simulink model "dspsdadc_sg_LL03_IIR_DC_rem"  (R2016b)
settings: Solver=ode5  StartTime=0.0  StopTime=2*pi*200000/2.4e6  MaxStep=1/512000  RelTol=1e-3  AbsTol=1e-6
PreLoadFcn:
  | input_rate = 2.5e6;
  | input_period = 1/input_rate;
  | decimation_factor = 64;
  | 
  | 
  | ila_PDM_data = read_vectored_ILA_PDM_capture('.\ILA_capture\iladata_A440_vectors_1024.csv');
  | % ila_PDM_data = read_vectored_ILA_PDM_capture('.\ILA_capture\iladata_speech_vectors_1024.csv');
  | 
  | ila_data_struct.time = [];
  | ila_data_struct.signals.values = ila_PDM_data;
  | 
  | % Delay parameter for IIR DC-removal filter
  | D= 256;
StopFcn:
  | p = audioplayer(squeeze(simout_demodulated_SG.Data), input_rate/decimation_factor);
  | play(p, [1 (get(p, 'SampleRate') * 1)]);
  | 
  | p = audioplayer(squeeze(simout_demodulated_FP.Data), input_rate/decimation_factor);
  | play(p, [1 (get(p, 'SampleRate') * 1)]);
undefined symbols (not defined in the file or in its folder): xlfda_numerator
libraries: xbsIndex_r4 x30, dspmlti4 x2, simulink x1, dspmisc x1
settings Model: ExtModeTrigMode=oneshot  ExtModeArmWhenConnect=off  ExtModeAutoUpdateStatusClock=off  Creator=The MathWorks Inc.  LastModifiedBy=Luc
settings DataIOCC: SaveFormat=Array  SaveOutput=off  SaveTime=off  SignalLoggingName=logsOut
settings OptimizationCC: BlockReduction=off  BooleanDataType=off  ExpressionDepthLimit=2147483647  RollThreshold=2  InitFltsAndDblsToZero=on  EfficientMapNaN2IntZero=off  LifeSpan=inf
settings DebuggingCC: SaveWithParameterizedLinksMsg=none  UnderspecifiedInitializationDetection=Classic  MergeDetectMultiDrivingBlocksExec=none  SignalResolutionControl=TryResolveAllWithWarning  MultiTaskDSMMsg=warning  MultiTaskCondExecSysMsg=none  IntegerOverflowMsg=none  FcnCallInpInsideContextMsg=warning  StateNameClashWarn=warning  SFUnexpectedBacktrackingDiag=warning  SFNoUnconditionalDefaultTransitionDiag=warning  SFExecutionAtInitializationDiag=none  IntegerSaturationMsg=none
settings HardwareCC: ProdBitPerPointer=32  ProdBitPerSizeT=32  ProdBitPerPtrDiffT=32  ProdLargestAtomicFloat=None  ProdIntDivRoundTo=Undefined  ProdEndianess=Unspecified  ProdWordSize=32  ProdHWDeviceType=32-bit Generic  TargetUnknown=on
settings ModelReferenceCC: PropagateSignalLabelsOutOfModel=off
settings GRTTargetCC: TargetFcnLib=ansi_tfl_tmw.mat  TargetLangStandard=C89/C90 (ANSI)  GeneratePreprocessorConditionals=Disable all  CombineOutputUpdateFcns=off  GRTInterface=on
settings ConfigComp: CovMetricSettings=dw  CovHtmlReporting=on  CovSaveCumulativeToWorkspaceVar=on  CovSaveSingleToWorkspaceVar=on  CovExternalEMLEnable=off

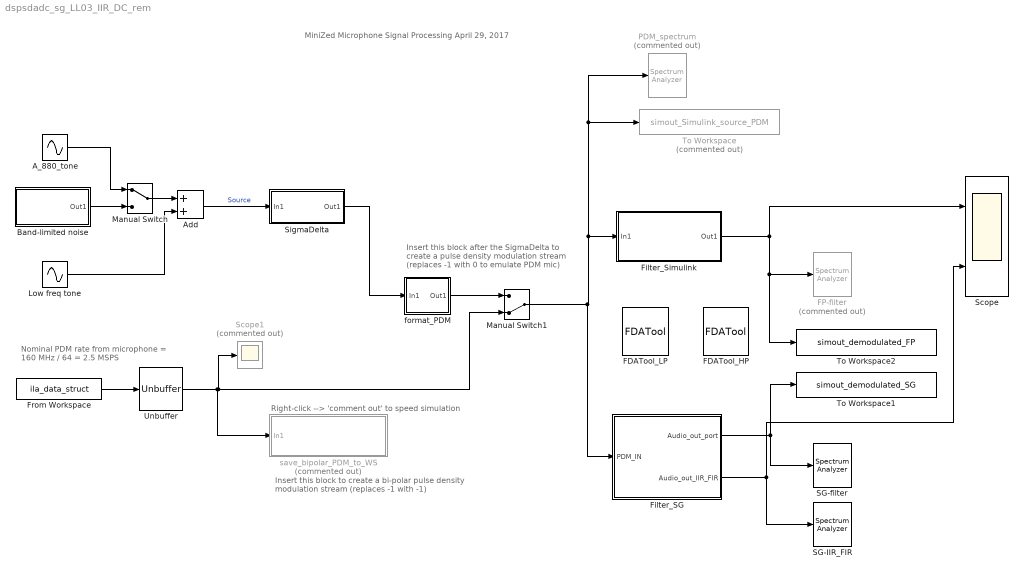
== system dspsdadc_sg_LL03_IIR_DC_rem ==
  note: Insert this block after the SigmaDelta to
      | create a pulse density modulation stream
      | (replaces -1 with 0 to emulate PDM mic)
  note: Insert this block to
      | create a bi-polar pulse density modulation stream
      | (replaces -1 with -1)
  note: Right-click --> 'comment out' to speed simulation
  note: Nominal PDM rate from microphone = 160 MHz / 64 = 2.5 MSPS
  note: MiniZed Microphone Signal Processing
      | April 29, 2017
  A_880_tone : Sin  Amplitude=0.5  Frequency=2*pi*880  SampleTime=input_period
  Add : Sum
  Band-limited noise : Subsystem
  FDATool_HP : xbsIndex_r4/FDATool  block_type=fdatool
      settings: infoedit=FDATool
  FDATool_LP : xbsIndex_r4/FDATool  block_type=fdatool
      settings: infoedit=FDATool
  FP-filter : SpectrumAnalyzer  Commented=on
  Filter_SG : Subsystem
  Filter_Simulink : Subsystem
  From Workspace : FromWorkspace  VariableName=ila_data_struct  OutDataTypeStr=double  SampleTime=input_period*1024  Interpolate=off  OutputAfterFinalValue=Cyclic repetition
  Low freq tone : Sin  Amplitude=0.0  Frequency=2*pi*5  SampleTime=input_period
  Manual Switch : ManualSwitch
  Manual Switch1 : ManualSwitch  CurrentSetting=0
  PDM_spectrum : SpectrumAnalyzer  Commented=on
  SG-IIR_FIR : SpectrumAnalyzer
  SG-filter : SpectrumAnalyzer
  Scope : Scope  NumInputPorts=2
  Scope1 : Scope  Commented=on
  SigmaDelta : Subsystem
  To Workspace : ToWorkspace  Commented=on  VariableName=simout_Simulink_source_PDM  SaveFormat=Timeseries  SampleTime=-1
  To Workspace1 : ToWorkspace  VariableName=simout_demodulated_SG  SaveFormat=Timeseries  SampleTime=-1
  To Workspace2 : ToWorkspace  VariableName=simout_demodulated_FP  SaveFormat=Timeseries  SampleTime=-1
  Unbuffer : Unbuffer  SampleBasedProcessing=Same as frame based
  format_PDM : Subsystem
  save_bipolar_PDM_to_WS : Subsystem  Commented=on
  wires:
  Add/1 -> SigmaDelta/1(In1)  "Source"
  Filter_SG/1(Audio_out_port) -> SG-filter/1, To Workspace1/1
  Filter_Simulink/1(Out1) -> Scope/1, To Workspace2/1, FP-filter/1
  Low freq tone/1 -> Add/2
  Manual Switch/1 -> Add/1
  A_880_tone/1 -> Manual Switch/1
  Band-limited noise/1(Out1) -> Manual Switch/2
  SigmaDelta/1(Out1) -> format_PDM/1(In1)
  Manual Switch1/1 -> PDM_spectrum/1, To Workspace/1, Filter_Simulink/1(In1), Filter_SG/1(PDM_IN)
  format_PDM/1(Out1) -> Manual Switch1/1
  From Workspace/1 -> Unbuffer/1
  Unbuffer/1 -> save_bipolar_PDM_to_WS/1(In1), Scope1/1, Manual Switch1/2
  Filter_SG/2(Audio_out_IIR_FIR) -> Scope/2, SG-IIR_FIR/1

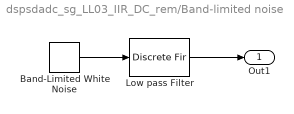
== system dspsdadc_sg_LL03_IIR_DC_rem/Band-limited noise ==
  Band-Limited White Noise : simulink/Sources/Band-Limited White Noise  Cov=[0.000001]  Ts=input_period  seed=[23341]
  Low pass Filter : DiscreteFir  Coefficients=xlfda_numerator([bdroot '/FDATool_LP'])
  Out1 : Outport
  wires:
  Band-Limited White Noise/1 -> Low pass Filter/1
  Low pass Filter/1 -> Out1/1

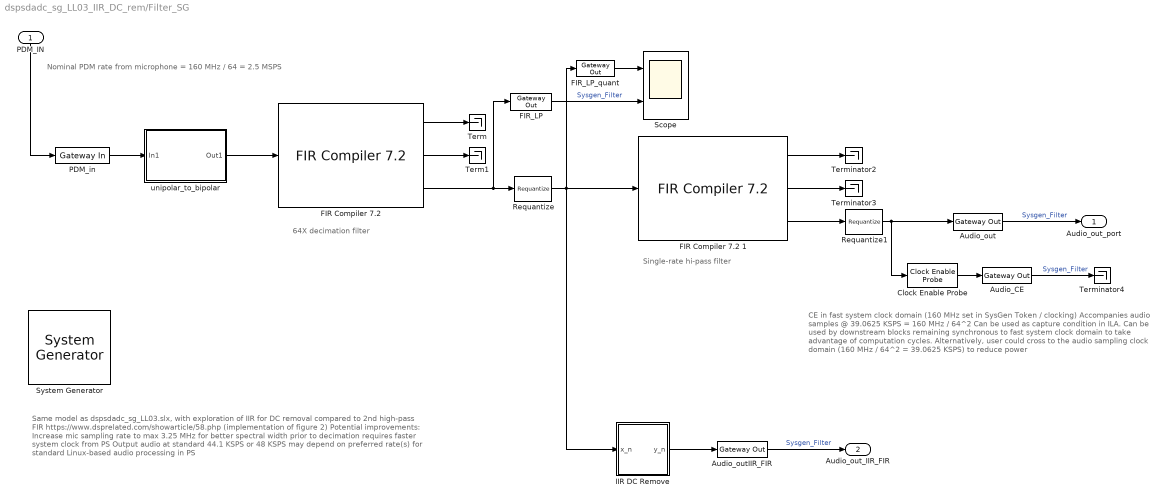
== system dspsdadc_sg_LL03_IIR_DC_rem/Filter_SG ==
  note: CE in fast system clock domain (160 MHz set in SysGen Token / clocking)
      | Accompanies audio samples @ 39.0625 KSPS = 160 MHz / 64^2
      |
      | Can be used as capture condition in ILA.
      |
      | Can be used by downstream blocks remaining synchronous to fast system clock domain to take advantage of computation cycles.
      |
      | Alternatively, user could cross to the audio sampling clock domain (160 MHz / 64^2 = 39.0625 KSPS) to reduce power
  note: Nominal PDM rate from microphone = 160 MHz / 64 = 2.5 MSPS
  note: 64X decimation filter
  note: Single-rate hi-pass filter
  note: Same model as dspsdadc_sg_LL03.slx, with exploration of IIR for DC removal compared to 2nd high-pass FIR
      | https://www.dsprelated.com/showarticle/58.php
      | (implementation of figure 2)
      |
      | Potential improvements:
      |
      | Increase mic sampling rate to max 3.25 MHz for better spectral width prior to decimation
      | requires faster system clock from PS
      | Output audio at standard 44.1 KSPS or 48 KSPS
      | may depend on preferred rate(s) for standard Linux-based audio processing in PS
  PDM_IN : Inport
  " System Generator" : xbsIndex_r4/ System Generator  Tag=genX  xilinxfamily=zynq  part=xc7z010  speed=-1  package=clg400  synthesis_tool=Vivado  clock_wrapper=Clock Enables  directory=C:/VivadoProjects/MiniZedBasic/SysGen/netlist  proj_type=Vivado  Synth_file=Vivado Synthesis Defaults  Impl_file=Vivado Implementation Defaults  testbench=off  simulink_period=1/(64*2.5e6)  sysclk_period=6.25  dcm_input_clock_period=10  incr_netlist=off  trim_vbits=Everywhere in SubSystem  dbl_ovrd=According to Block Masks  core_generation=According to Block Masks  run_coregen=off  deprecated_control=off  eval_field=0  block_type=sysgen
  Audio_CE : xbsIndex_r4/Gateway Out  inherit_from_input=off  hdl_port=on  rows=1  columns=1  UseAsDAC=off  DACChannel='1'  interface=None  automatic_assignment=on  address_offset=hex2dec('00')  intf_name=''  intf_description=''  timing_constraint=None  locs_specified=off  LOCs={}  io_standard={}  block_type=gatewayout
  Audio_out : xbsIndex_r4/Gateway Out  inherit_from_input=off  hdl_port=on  rows=1  columns=1  UseAsDAC=off  DACChannel='1'  interface=None  automatic_assignment=on  address_offset=hex2dec('00')  intf_name=''  intf_description=''  timing_constraint=None  locs_specified=off  LOCs={}  io_standard={}  block_type=gatewayout
  Audio_outIIR_FIR : xbsIndex_r4/Gateway Out  inherit_from_input=off  hdl_port=on  rows=1  columns=1  UseAsDAC=off  DACChannel='1'  interface=None  automatic_assignment=on  address_offset=hex2dec('00')  intf_name=''  intf_description=''  timing_constraint=None  locs_specified=off  LOCs={}  io_standard={}  block_type=gatewayout
  Clock Enable Probe : xbsIndex_r4/Clock Enable Probe  inherit_constraints=off  block_type=ceprobe
      settings: infoedit="Clock enable extractor.  Produces a Boolean output that mirrors the hardware clock enable associated with the input sample rate.<br><br>Hardware notes: in hardware this block costs nothing."
  "FIR Compiler 7.2 " : xbsIndex_r4/FIR Compiler 7.2   coefficientvector=xlfda_numerator([bdroot '/FDATool_LP'])* decimation_factor  coefficient_sets=1  coefficient_reload=off  filter_type=Decimation  rate_change_type=Integer  interpolation_rate=1  decimation_rate=decimation_factor  zero_pack_factor=1  channel_sequence=Basic  number_channels=1  pattern_list='P4-0,P4-1,P4-2,P4-3,P4-4'  number_paths=1  ratespecification=Maximum_Possible  sampleperiod=4096  hardwareoversamplingrate=1  coefficient_sign=Signed  quantization=Maximize_Dynamic_Range  coefficient_width=16  bestprecision=on  coefficient_fractional_bits=15  coefficient_structure=Symmetric  output_rounding_mode=Symmetric_Rounding_to_Infinity  output_width=21  filter_architecture=Systolic_Multiply_Accumulate  optimization_goal=Area  optimization_list='None'  data_buffer_type=Automatic  coefficient_buffer_type=Automatic  input_buffer_type=Automatic  output_buffer_type=Automatic  preference_for_other_storage=Automatic  multi_column_support=Automatic  columnconfig='10'  inter_column_pipe_length=4  data_has_tlast=Not_Required  m_data_has_tready=off  s_data_has_fifo=off  s_data_has_tuser=Not_Required  m_data_has_tuser=Not_Required  s_config_sync_mode=On_Vector  s_config_method=Single  num_reload_slots=1  has_aclken=off  has_aresetn=off  infoeditControl=ARESETn must be asserted for a minimum of 2 cycles  reset_data_vector=on  trim_axipin_name=on  simulation_type=hybrid_sim  simulation_model=sysgen:xfirv7_2_cmodel  data_path_portlist={ 's_axis_data_tdata', 'm_axis_data_tdata' }  passband_min=0.0  passband_max=0.5  stopband_min=0.5  stopband_max=1.0  filter_selection=1  gui_behaviour='Sysgen_GUI'  data_sign=Signed  data_width=16  data_fractional_bits=0  data_tuser_width=1  wrapper_available=true  ip_wrap_arbitrary_binary_point=true  ip_name=FIR Compiler  ip_version=7.2  dsptool_ready=true  ipcore_usecache=true  ipcore_useipmodelcache=true  port_translation_map={ 'aclken' => 'en', 'aresetn' => 'rst' }  run_core_at_system_period=true  ipcore_xco_need_fpga_part=true  block_type=fir_compiler_v7_2
      settings: infoedit=Maximum Possible : Maximizes oversampling rate. Abstracted input handshake (no s_data_tvalid) and automatic rate propagation.<br>Hardware Oversampling Rate : Specifies oversampling rate relative to the input sample period. Abstracted input handshake (no s_data_tvalid) and automatic rate propagation.<br>Input/Output Sample Period : Specifies absolute oversampling rate. No input handshake abstraction (exposes s_data_tvalid) and no rate propagation.
  FIR Compiler 7.2 1 : xbsIndex_r4/FIR Compiler 7.2   coefficientvector=xlfda_numerator([bdroot '/FDATool_HP'])  coefficient_sets=1  coefficient_reload=off  filter_type=Single_Rate  rate_change_type=Integer  interpolation_rate=1  decimation_rate=1  zero_pack_factor=1  channel_sequence=Basic  number_channels=1  pattern_list='P4-0,P4-1,P4-2,P4-3,P4-4'  number_paths=1  ratespecification=Maximum_Possible  sampleperiod=4096  hardwareoversamplingrate=1  coefficient_sign=Signed  quantization=Maximize_Dynamic_Range  coefficient_width=16  bestprecision=on  coefficient_fractional_bits=15  coefficient_structure=Symmetric  output_rounding_mode=Symmetric_Rounding_to_Infinity  output_width=15  filter_architecture=Systolic_Multiply_Accumulate  optimization_goal=Area  optimization_list='None'  data_buffer_type=Automatic  coefficient_buffer_type=Automatic  input_buffer_type=Automatic  output_buffer_type=Automatic  preference_for_other_storage=Automatic  multi_column_support=Automatic  columnconfig='40,40'  inter_column_pipe_length=4  data_has_tlast=Not_Required  m_data_has_tready=off  s_data_has_fifo=off  s_data_has_tuser=Not_Required  m_data_has_tuser=Not_Required  s_config_sync_mode=On_Vector  s_config_method=Single  num_reload_slots=1  has_aclken=off  has_aresetn=off  infoeditControl=ARESETn must be asserted for a minimum of 2 cycles  reset_data_vector=on  trim_axipin_name=on  simulation_type=hybrid_sim  simulation_model=sysgen:xfirv7_2_cmodel  data_path_portlist={ 's_axis_data_tdata', 'm_axis_data_tdata' }  passband_min=0.0  passband_max=0.5  stopband_min=0.5  stopband_max=1.0  filter_selection=1  gui_behaviour='Sysgen_GUI'  data_sign=Signed  data_width=16  data_fractional_bits=0  data_tuser_width=1  wrapper_available=true  ip_wrap_arbitrary_binary_point=true  ip_name=FIR Compiler  ip_version=7.2  dsptool_ready=true  ipcore_usecache=true  ipcore_useipmodelcache=true  port_translation_map={ 'aclken' => 'en', 'aresetn' => 'rst' }  run_core_at_system_period=true  ipcore_xco_need_fpga_part=true  block_type=fir_compiler_v7_2
      settings: infoedit=Maximum Possible : Maximizes oversampling rate. Abstracted input handshake (no s_data_tvalid) and automatic rate propagation.<br>Hardware Oversampling Rate : Specifies oversampling rate relative to the input sample period. Abstracted input handshake (no s_data_tvalid) and automatic rate propagation.<br>Input/Output Sample Period : Specifies absolute oversampling rate. No input handshake abstraction (exposes s_data_tvalid) and no rate propagation.
  FIR_LP : xbsIndex_r4/Gateway Out  inherit_from_input=off  hdl_port=off  rows=1  columns=1  UseAsDAC=off  DACChannel='1'  interface=None  automatic_assignment=on  address_offset=hex2dec('00')  intf_name=''  intf_description=''  timing_constraint=None  locs_specified=off  LOCs={}  io_standard={}  block_type=gatewayout
  FIR_LP_quant : xbsIndex_r4/Gateway Out  inherit_from_input=off  hdl_port=off  rows=1  columns=1  UseAsDAC=off  DACChannel='1'  interface=None  automatic_assignment=on  address_offset=hex2dec('00')  intf_name=''  intf_description=''  timing_constraint=None  locs_specified=off  LOCs={}  io_standard={}  block_type=gatewayout
  IIR DC Remove : Subsystem
  PDM_in : xbsIndex_r4/Gateway In  gui_display_data_type=Boolean  arith_type=Boolean  n_bits=1  bin_pt=0  preci_type=Single  exp_width=8  frac_width=24  rows=1  columns=1  quantization=Truncate  overflow=Flag as error  period=1/input_rate  UseAsADC=off  ADCChannel='1'  interface=None  automatic_assignment=on  address_offset=hex2dec('00')  intf_name=''  intf_description=''  default_value=0  timing_constraint=None  locs_specified=off  LOCs={}  io_standard={}  inherit_from_input=off  hdl_port=on  dbl_ovrd=off  block_type=gatewayin
  Requantize : xbsIndex_r4/Requantize  scale_factor=0  n_bits=14  bin_pt=11  simulation_type=fast_sim  simulation_model=sysgen:requantizer  block_type=requantizer
  Requantize1 : xbsIndex_r4/Requantize  scale_factor=0  n_bits=16  bin_pt=13  simulation_type=fast_sim  simulation_model=sysgen:requantizer  block_type=requantizer
  Scope : Scope  NumInputPorts=2
  Term : Terminator
  Term1 : Terminator
  Terminator2 : Terminator
  Terminator3 : Terminator
  Terminator4 : Terminator
  unipolar_to_bipolar : Subsystem
  Audio_out_port : Outport
  Audio_out_IIR_FIR : Outport  Port=2
  wires:
  Audio_out/1 -> Audio_out_port/1  "Sysgen_Filter"
  "FIR Compiler 7.2 "/1 -> Term/1
  "FIR Compiler 7.2 "/2 -> Term1/1
  PDM_IN/1 -> PDM_in/1
  PDM_in/1 -> unipolar_to_bipolar/1(In1)
  "FIR Compiler 7.2 "/3 -> FIR_LP/1, Requantize/1
  FIR Compiler 7.2 1/1 -> Terminator2/1
  FIR Compiler 7.2 1/2 -> Terminator3/1
  FIR Compiler 7.2 1/3 -> Requantize1/1
  Clock Enable Probe/1 -> Audio_CE/1
  Audio_CE/1 -> Terminator4/1  "Sysgen_Filter"
  unipolar_to_bipolar/1(Out1) -> "FIR Compiler 7.2 "/1
  Requantize/1 -> IIR DC Remove/1(x_n), FIR_LP_quant/1, FIR Compiler 7.2 1/1
  Requantize1/1 -> Clock Enable Probe/1, Audio_out/1
  FIR_LP_quant/1 -> Scope/1
  FIR_LP/1 -> Scope/2  "Sysgen_Filter"
  Audio_outIIR_FIR/1 -> Audio_out_IIR_FIR/1  "Sysgen_Filter"
  IIR DC Remove/1(y_n) -> Audio_outIIR_FIR/1

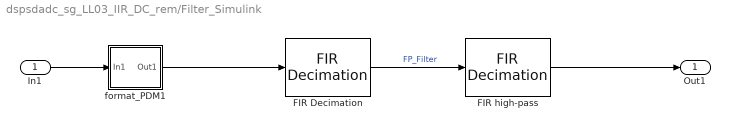
== system dspsdadc_sg_LL03_IIR_DC_rem/Filter_Simulink ==
  In1 : Inport
  FIR Decimation : dspmlti4/FIR Decimation  FilterSource=Dialog parameters  h=xlfda_numerator([bdroot '/FDATool_LP'])  D=decimation_factor  filtStruct=Direct form  FilterObject=Hm_firdecim  InputProcessing=Columns as channels (frame based)  framing=Allow multirate processing  inputOffset=0  outputBufInitCond=0  roundingMode=Floor  overflowMode=off  firstCoeffDataTypeStr=Inherit: Same word length as input  firstCoeffMin=[]  firstCoeffMax=[]  firstCoeffLastDataTypeStr=Inherit: Same word length as input  outputDataTypeStr=Inherit: Same as accumulator  outputMin=[]  outputMax=[]  outputLastDataTypeStr=Inherit: Same as accumulator
  "FIR high-pass " : dspmlti4/FIR Decimation  FilterSource=Dialog parameters  h=xlfda_numerator([bdroot '/FDATool_HP'])  D=1  filtStruct=Direct form  FilterObject=Hm_firdecim  InputProcessing=Columns as channels (frame based)  framing=Allow multirate processing  inputOffset=0  outputBufInitCond=0  roundingMode=Floor  overflowMode=off  firstCoeffDataTypeStr=Inherit: Same word length as input  firstCoeffMin=[]  firstCoeffMax=[]  firstCoeffLastDataTypeStr=Inherit: Same word length as input  outputDataTypeStr=Inherit: Same as accumulator  outputMin=[]  outputMax=[]  outputLastDataTypeStr=Inherit: Same as accumulator
  format_PDM1 : Subsystem
  Out1 : Outport
  wires:
  FIR Decimation/1 -> "FIR high-pass "/1  "FP_Filter"
  In1/1 -> format_PDM1/1(In1)
  "FIR high-pass "/1 -> Out1/1
  format_PDM1/1(Out1) -> FIR Decimation/1

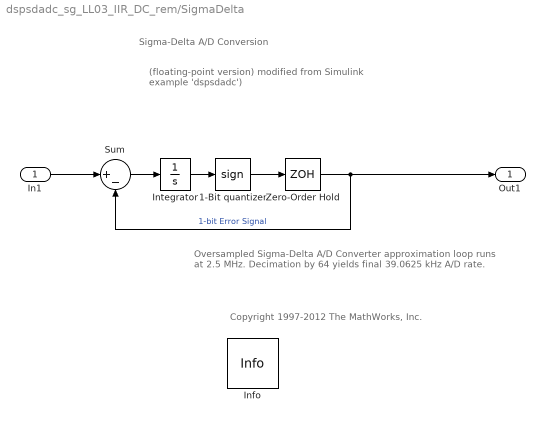
== system dspsdadc_sg_LL03_IIR_DC_rem/SigmaDelta ==
  note: Oversampled Sigma-Delta A/D Converter
      | approximation loop runs at 2.5 MHz.
      | Decimation by 64 yields final 39.0625 kHz A/D rate.
  note: Copyright 1997-2012 The MathWorks, Inc.
  note: Sigma-Delta A/D Conversion
  note: (floating-point version)
      | modified from Simulink example 'dspsdadc')
  In1 : Inport
  1-Bit quantizer : Signum
  Info : dspmisc/Info  SystemSampleTime=-1
  Integrator : Integrator
  Sum : Sum  Inputs=|+-  SaturateOnIntegerOverflow=on  InputSameDT=on  OutDataTypeStr=Inherit: Same as first input
  Zero-Order Hold : ZeroOrderHold  SampleTime=input_period
  Out1 : Outport
  wires:
  Zero-Order Hold/1 -> Out1/1, Sum/2  "1-bit Error Signal"
  1-Bit quantizer/1 -> Zero-Order Hold/1
  Sum/1 -> Integrator/1
  Integrator/1 -> 1-Bit quantizer/1
  In1/1 -> Sum/1

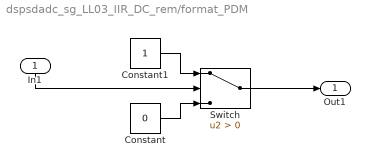
== system dspsdadc_sg_LL03_IIR_DC_rem/format_PDM ==
  In1 : Inport
  Constant : Constant  Value=0
  Constant1 : Constant
  Switch : Switch  Criteria=u2 > Threshold
  Out1 : Outport
  wires:
  In1/1 -> Switch/2
  Constant1/1 -> Switch/1
  Constant/1 -> Switch/3
  Switch/1 -> Out1/1

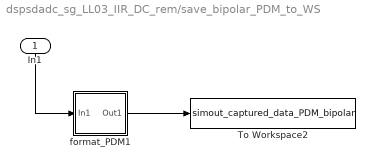
== system dspsdadc_sg_LL03_IIR_DC_rem/save_bipolar_PDM_to_WS ==
  In1 : Inport
  To Workspace2 : ToWorkspace  VariableName=simout_captured_data_PDM_bipolar  SaveFormat=Timeseries  SampleTime=-1
  format_PDM1 : Subsystem
  wires:
  In1/1 -> format_PDM1/1(In1)
  format_PDM1/1(Out1) -> To Workspace2/1

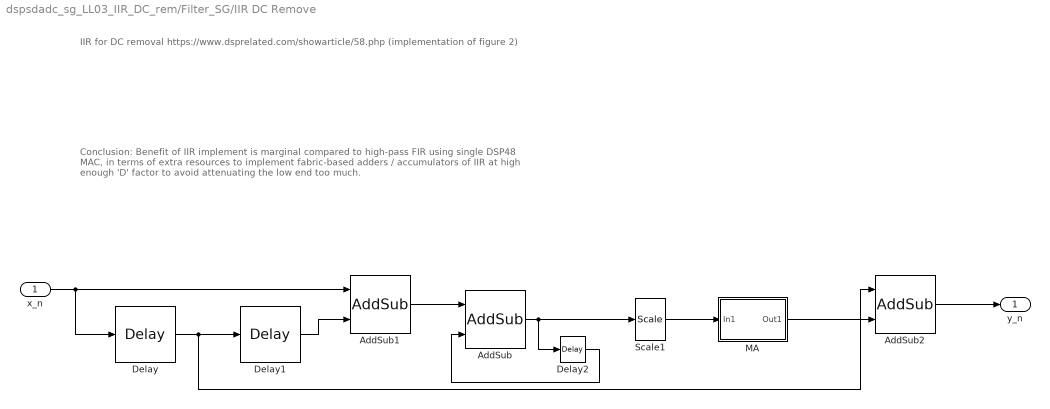
== system dspsdadc_sg_LL03_IIR_DC_rem/Filter_SG/IIR DC Remove ==
  note: IIR for DC removal
      | https://www.dsprelated.com/showarticle/58.php
      | (implementation of figure 2)
  note: Conclusion:
      | Benefit of IIR implement is marginal compared to high-pass FIR using single DSP48 MAC, in terms of extra resources to implement fabric-based adders / accumulators of IIR at high enough 'D' factor to avoid attenuating the low end too much.
  x_n : Inport
  AddSub : xbsIndex_r4/AddSub  mode=Addition  use_carryin=off  use_carryout=off  en=off  latency=0  precision=User Defined  arith_type="Signed  (2's comp)"  n_bits=log2(D)+15  bin_pt=11  quantization=Truncate  overflow=Flag as error  use_behavioral_HDL=off  hw_selection=Fabric  pipelined=off  dbl_ovrd=off  block_type=addsub
  AddSub1 : xbsIndex_r4/AddSub  mode=Subtraction  use_carryin=off  use_carryout=off  en=off  latency=0  precision=Full  arith_type="Signed  (2's comp)"  n_bits=3  bin_pt=0  quantization=Truncate  overflow=Wrap  use_behavioral_HDL=off  hw_selection=Fabric  pipelined=off  dbl_ovrd=off  block_type=addsub
  AddSub2 : xbsIndex_r4/AddSub  mode=Subtraction  use_carryin=off  use_carryout=off  en=off  latency=1  precision=Full  arith_type=Unsigned  n_bits=16  bin_pt=14  quantization=Truncate  overflow=Wrap  use_behavioral_HDL=off  hw_selection=Fabric  pipelined=off  dbl_ovrd=off  block_type=addsub
  Delay : xbsIndex_r4/Delay  rst=off  infoeditControl=Selection of Reset will increase slice count due to use of real FFs and instead of SRLs  en=off  latency=D-1  reg_retiming=off  dbl_ovrd=off  block_type=delay
  Delay1 : xbsIndex_r4/Delay  rst=off  infoeditControl=Selection of Reset will increase slice count due to use of real FFs and instead of SRLs  en=off  latency=1  reg_retiming=off  dbl_ovrd=off  block_type=delay
  Delay2 : xbsIndex_r4/Delay  rst=off  infoeditControl=Selection of Reset will increase slice count due to use of real FFs and instead of SRLs  en=off  latency=1  reg_retiming=off  dbl_ovrd=off  block_type=delay
  MA : Subsystem
  Scale1 : xbsIndex_r4/Scale  scale_factor=-log2(D)  dbl_ovrd=off  block_type=scale
  y_n : Outport
  wires:
  AddSub1/1 -> AddSub/1
  x_n/1 -> Delay/1, AddSub1/1
  Delay/1 -> AddSub2/1, Delay1/1
  AddSub/1 -> Delay2/1, Scale1/1
  MA/1(Out1) -> AddSub2/2
  AddSub2/1 -> y_n/1
  Delay1/1 -> AddSub1/2
  Delay2/1 -> AddSub/2
  Scale1/1 -> MA/1(In1)

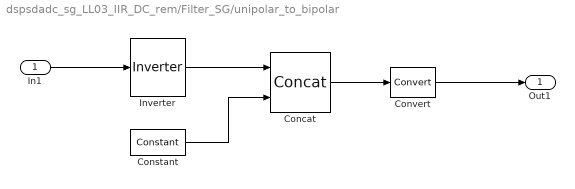
== system dspsdadc_sg_LL03_IIR_DC_rem/Filter_SG/unipolar_to_bipolar ==
  In1 : Inport
  Concat : xbsIndex_r4/Concat  num_inputs=2  dbl_ovrd=off  block_type=concat
  Constant : xbsIndex_r4/Constant  const=1.0  gui_display_data_type=Boolean  arith_type=Boolean  n_bits=16  bin_pt=14  preci_type=Single  exp_width=8  frac_width=24  explicit_period=off  period=1  equ=P=C  opselect=C  inp2=PCIN>>17  opr=+  inp1=P  carry=CIN  dbl_ovrd=off  block_type=constant
  Convert : xbsIndex_r4/Convert  gui_display_data_type=Fixed-point  arith_type="Signed  (2's comp)"  n_bits=2  bin_pt=0  float_type=Single  exp_bits=8  fraction_bits=24  quantization=Truncate  overflow=Wrap  en=off  latency=1  pipeline=off  dbl_ovrd=off  block_type=convert
  Inverter : xbsIndex_r4/Inverter  en=off  latency=1  dbl_ovrd=off  block_type=inv
  Out1 : Outport
  wires:
  Constant/1 -> Concat/2
  Inverter/1 -> Concat/1
  In1/1 -> Inverter/1
  Convert/1 -> Out1/1
  Concat/1 -> Convert/1

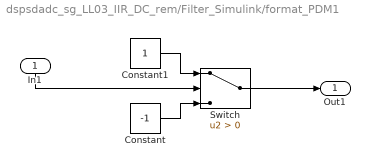
== system dspsdadc_sg_LL03_IIR_DC_rem/Filter_Simulink/format_PDM1 ==
  In1 : Inport
  Constant : Constant  Value=-1
  Constant1 : Constant
  Switch : Switch  Criteria=u2 > Threshold
  Out1 : Outport
  wires:
  In1/1 -> Switch/2
  Constant1/1 -> Switch/1
  Constant/1 -> Switch/3
  Switch/1 -> Out1/1

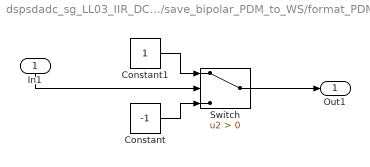
== system dspsdadc_sg_LL03_IIR_DC_rem/save_bipolar_PDM_to_WS/format_PDM1 ==
  In1 : Inport
  Constant : Constant  Value=-1
  Constant1 : Constant
  Switch : Switch  Criteria=u2 > Threshold
  Out1 : Outport
  wires:
  In1/1 -> Switch/2
  Constant1/1 -> Switch/1
  Constant/1 -> Switch/3
  Switch/1 -> Out1/1

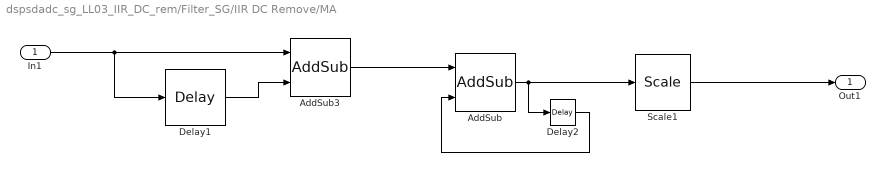
== system dspsdadc_sg_LL03_IIR_DC_rem/Filter_SG/IIR DC Remove/MA ==
  In1 : Inport
  AddSub : xbsIndex_r4/AddSub  mode=Addition  use_carryin=off  use_carryout=off  en=off  latency=0  precision=User Defined  arith_type="Signed  (2's comp)"  n_bits=log2(D)+21  bin_pt=19  quantization=Truncate  overflow=Flag as error  use_behavioral_HDL=off  hw_selection=Fabric  pipelined=off  dbl_ovrd=off  block_type=addsub
  AddSub3 : xbsIndex_r4/AddSub  mode=Subtraction  use_carryin=off  use_carryout=off  en=off  latency=0  precision=Full  arith_type="Signed  (2's comp)"  n_bits=10  bin_pt=log2(D)  quantization=Truncate  overflow=Flag as error  use_behavioral_HDL=off  hw_selection=Fabric  pipelined=off  dbl_ovrd=off  block_type=addsub
  Delay1 : xbsIndex_r4/Delay  rst=off  infoeditControl=Selection of Reset will increase slice count due to use of real FFs and instead of SRLs  en=off  latency=D  reg_retiming=off  dbl_ovrd=off  block_type=delay
  Delay2 : xbsIndex_r4/Delay  rst=off  infoeditControl=Selection of Reset will increase slice count due to use of real FFs and instead of SRLs  en=off  latency=1  reg_retiming=off  dbl_ovrd=off  block_type=delay
  Scale1 : xbsIndex_r4/Scale  scale_factor=-log2(D)  dbl_ovrd=off  block_type=scale
  Out1 : Outport
  wires:
  In1/1 -> Delay1/1, AddSub3/1
  Scale1/1 -> Out1/1
  AddSub3/1 -> AddSub/1
  Delay1/1 -> AddSub3/2
  AddSub/1 -> Scale1/1, Delay2/1
  Delay2/1 -> AddSub/2
